simulink model "dc_motor_control_MIO_16E4_2015a"  (R2015a)
settings: Solver=ode3  SolverMode=SingleTasking  StartTime=0.0  StopTime=2  RelTol=1e-3
model workspace (MAT data in the model file):
  freq = 0
  tau = 0
values from neighbouring files (symbols this model uses):
  a = 37.04    [ControlSystemDesigner_e_Nyquist.m]    (also in ex3_5.m)
  k0 = 1.382    [ControlSystemDesigner_e_Nyquist.m]
  k1 = 6.9094    [ControlSystemDesigner_e_Nyquist.m]
  z = 14.89    [ControlSystemDesigner_e_Nyquist.m]    (also in ex3_5.m = 5)
undefined symbols (not defined in the file or in its folder): MIO, National_Instruments, PCI
libraries: sldrtlib x5
settings Model: SimulationMode=external  ExtModeTrigDuration=60001  Creator=Alunos  LastModifiedBy=alunos
settings OptimizationCC: BlockReduction=off  BooleanDataType=off
settings DebuggingCC: SaveWithParameterizedLinksMsg=none  UnderspecifiedInitializationDetection=Classic  MergeDetectMultiDrivingBlocksExec=none  SignalResolutionControl=TryResolveAllWithWarning
settings HardwareCC: ProdIntDivRoundTo=Zero  ProdEndianess=LittleEndian  ProdHWDeviceType=Intel->x86/Pentium  TargetIntDivRoundTo=Zero  TargetEndianess=LittleEndian  TargetHWDeviceType=Intel->x86/Pentium
settings RTWCC: SystemTargetFile=rtwin.tlc  TemplateMakefile=rtwin.tmf  Description=Simulink Desktop Real-Time  RTWCompilerOptimization=on
settings CodeAppCC: MaxIdLength=95
settings TargetCC: TargetPreCompLibLocation=C:\Program Files\MATLAB\R2015a\toolbox\sldrt\lib\win32

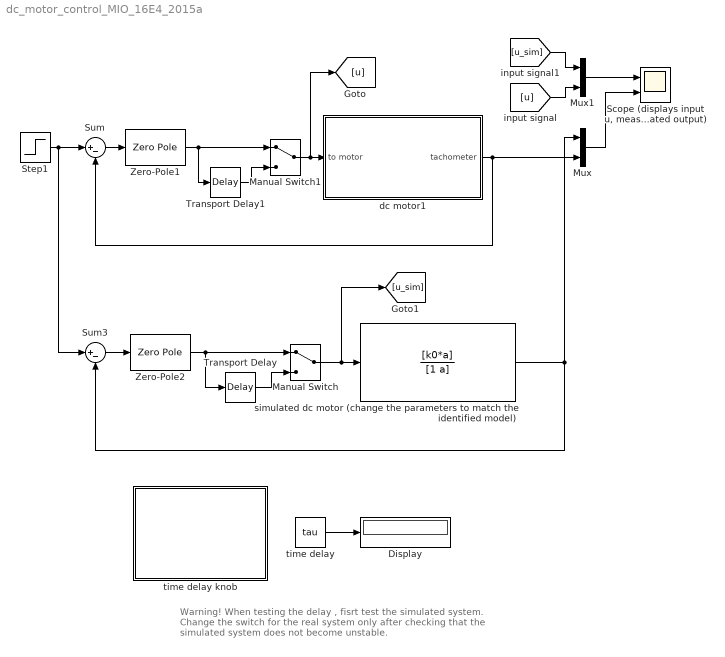
== system dc_motor_control_MIO_16E4_2015a ==
  note: Warning! When testing the delay , fisrt test the simulated system.
      | Change the switch for the real system only after checking
      | that the simulated system does not become unstable.
  Display : Display
  Manual Switch : ManualSwitch
  Manual Switch1 : ManualSwitch
  Mux : Mux  Inputs=2
  Mux1 : Mux  Inputs=2
  "Scope (displays input u, measured output, and simulated output)" : Scope  NumInputPorts=2
      settings: TimeRange=2  YMin=0~-0.2  YMax=2~1.2
  Step1 : Step  Time=0.2  SampleTime=0
  Sum : Sum  Inputs=|+-
  Sum3 : Sum  Inputs=|+-
  Transport Delay : TransportDelay  DelayTime=tau  FixedBuffer=on  TransDelayFeedthrough=on
  Transport Delay1 : TransportDelay  DelayTime=tau  InitialOutput=26.5714  FixedBuffer=on  TransDelayFeedthrough=on
  Zero-Pole1 : ZeroPole  Zeros=[-z]  Poles=[0]  Gain=[k1/z]
  Zero-Pole2 : ZeroPole  Zeros=[-z]  Poles=[0]  Gain=[k1/z]
  dc motor1 : Subsystem
  simulated dc motor (change the parameters to match the identified model) : TransferFcn  Numerator=[k0*a]  Denominator=[1 a]
  time delay : Constant  Value=tau
  time delay knob : Subsystem  DialogController=hmiCreateDDGDialog  IsWebBlock=on  mask(MathWorksWebBlock){webBlockId=95d73932-2942-4144-b5cc-49e721721c50, webBlockType=continuousknob, ShowInLibBrowser=on, ShowInitialText=on, HMISrcModelName=dc_motor_control_MIO_16E4_2015a}
      mask prompts: webBlockId "WebBlock Id"; webBlockType "WebBlock Type"; HMISrcModelName "Source Model"
      mask Help: helpview([docroot '/mapfiles/simulink.map'], 'hmi_knob')
      mask Display:
      | if strcmp(get_param(bdroot(gcb),'BlockDiagramType'), 'library')
      |     image([(matlabroot) '/toolbox/simulink/hmi/icons/ContinuousKnob.png']);
      | end
  wires:
  Mux/1 -> "Scope (displays input u, measured output, and simulated output)"/2
  Sum/1 -> Zero-Pole1/1
  Zero-Pole2/1 -> Transport Delay/1, Manual Switch/1
  Mux1/1 -> "Scope (displays input u, measured output, and simulated output)"/1
  Step1/1 -> Sum3/1, Sum/1
  simulated dc motor (change the parameters to match the identified model)/1 -> Sum3/2, Mux/1
  Sum3/1 -> Zero-Pole2/1
  dc motor1/1(tachometer) -> Sum/2, Mux/2
  [u_sim] -> Mux1/1
  [u] -> Mux1/2
  Manual Switch/1 -> [u_sim], simulated dc motor (change the parameters to match the identified model)/1
  Transport Delay/1 -> Manual Switch/2
  Zero-Pole1/1 -> Manual Switch1/1, Transport Delay1/1
  Transport Delay1/1 -> Manual Switch1/2
  Manual Switch1/1 -> [u], dc motor1/1(to motor)
  time delay/1 -> Display/1

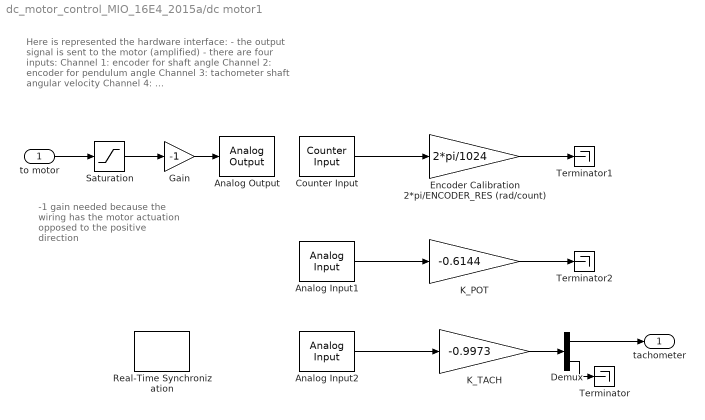
== system dc_motor_control_MIO_16E4_2015a/dc motor1 ==
  note: -1 gain needed
      | because the wiring
      | has the motor
      | actuation opposed to
      | the positive direction
  note: Here is represented the hardware interface:
      | - the output signal is sent to the motor (amplified)
      | - there are four inputs:
      | Channel 1: encoder for shaft angle
      | Channel 2: encoder for pendulum angle
      | Channel 3: tachometer shaft angular velocity
      | Channel 4: ...
  to motor : Inport
  Analog Input1 : sldrtlib/Analog Input  SampleTime=0.001  MaxMissedTicks=10  ShowMissedTicks=off  YieldWhenWaiting=off  DrvName=National_Instruments/PCI-MIO-16E-4  DrvAddress=4294967295  DrvOptions=[0 0 0 0 1 0]  Channels=1:2  RangeMode=1  VoltRange=1  DataType=1
      settings: AttributesFormatString=National Instruments\nPCI-MIO-16E-4 [auto]
  Analog Input2 : sldrtlib/Analog Input  SampleTime=0.001  MaxMissedTicks=10  ShowMissedTicks=off  YieldWhenWaiting=off  DrvName=National_Instruments/PCI-MIO-16E-4  DrvAddress=4294967295  DrvOptions=[0 0 0 0 1 0]  Channels=3:4  RangeMode=1  VoltRange=1  DataType=1
      settings: AttributesFormatString=National Instruments\nPCI-MIO-16E-4 [auto]
  Analog Output : sldrtlib/Analog Output  SampleTime=0.001  MaxMissedTicks=inf  ShowMissedTicks=off  YieldWhenWaiting=off  DrvName=National_Instruments/PCI-MIO-16E-4  DrvAddress=4294967295  DrvOptions=[0 0 0 0 1 0]  Channels=1  RangeMode=1  VoltRange=1  InitialValue=[]  FinalValue=0
      settings: AttributesFormatString=National Instruments\nPCI-MIO-16E-4 [auto]
  Counter Input : sldrtlib/Counter Input  SampleTime=0.001  MaxMissedTicks=inf  ShowMissedTicks=off  YieldWhenWaiting=off  DrvName=National_Instruments/PCI-MIO-16E-4  DrvAddress=4294967295  DrvOptions=[0 0 0 0 1 0]  Channels=1:2  ResetMode=1  CounterEdge=1  CounterGate=1  DataType=1
      settings: AttributesFormatString=National Instruments\nPCI-MIO-16E-4 [auto]
  Demux : Demux  Outputs=2
  Encoder Calibration 2*pi/ENCODER_RES (rad/count) : Gain  Gain=2*pi/1024  SaturateOnIntegerOverflow=on  OutDataTypeStr=Inherit: Same as input  ParamDataTypeStr=Inherit: Same as input
  Gain : Gain  Gain=-1
  K_POT : Gain  Gain=-0.6144  SaturateOnIntegerOverflow=on  OutDataTypeStr=Inherit: Same as input  ParamDataTypeStr=Inherit: Same as input
  "K_TACH " : Gain  Gain=-0.9973  SaturateOnIntegerOverflow=on  OutDataTypeStr=Inherit: Same as input  ParamDataTypeStr=Inherit: Same as input
  Real-Time Synchronization : sldrtlib/Real-Time Synchronization  SampleTime=0.001  MaxMissedTicks=inf  ShowMissedTicks=off  YieldWhenWaiting=off
  Saturation : Saturate  UpperLimit=10  LowerLimit=-10
  Terminator : Terminator
  Terminator1 : Terminator
  Terminator2 : Terminator
  tachometer : Outport
  wires:
  Analog Input1/1 -> K_POT/1
  Gain/1 -> Analog Output/1
  Counter Input/1 -> Encoder Calibration 2*pi/ENCODER_RES (rad/count)/1
  Analog Input2/1 -> "K_TACH "/1
  "K_TACH "/1 -> Demux/1
  Demux/1 -> tachometer/1
  Demux/2 -> Terminator/1
  to motor/1 -> Saturation/1
  Saturation/1 -> Gain/1
  Encoder Calibration 2*pi/ENCODER_RES (rad/count)/1 -> Terminator1/1
  K_POT/1 -> Terminator2/1

== system dc_motor_control_MIO_16E4_2015a/time delay knob ==
